simulink model "pmsm_foc_tune_2_2019"  (R2019b)
settings: Solver=VariableStepAuto  StartTime=0.0  StopTime=3  RelTol=1e-3
undefined symbols (not defined in the file): powergui
libraries: simulink x8, eePwmGenerator x6, powerlib x3
settings Model: Creator=ayanc  LastModifiedBy=ayanc

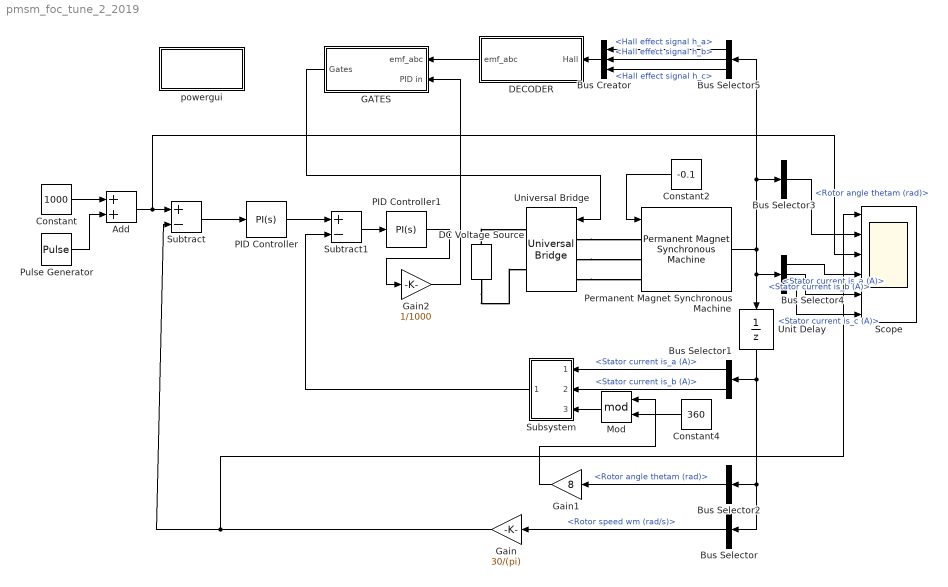
== system pmsm_foc_tune_2_2019 ==
  Add : Sum
  Bus Creator : BusCreator  Inputs=3
  Bus Selector : BusSelector  OutputSignals=Rotor speed wm (rad/s)
  Bus Selector1 : BusSelector  OutputSignals=Stator current is_a (A),Stator current is_b (A)
  Bus Selector2 : BusSelector  OutputSignals=Rotor angle thetam (rad)
  Bus Selector3 : BusSelector  OutputSignals=Rotor angle thetam (rad)
  Bus Selector4 : BusSelector  OutputSignals=Stator current is_a (A),Stator current is_b (A),Stator current is_c (A)
  Bus Selector5 : BusSelector  OutputSignals=Hall effect signal h_a,Hall effect signal h_b,Hall effect signal h_c
  Constant : Constant  Value=1000
  Constant2 : Constant  Value=-0.1
  Constant4 : Constant  Value=360
  DC Voltage Source : powerlib/Electrical Sources/DC Voltage Source  Amplitude=18  Measurements=None
  DECODER : Subsystem
  GATES : Subsystem
  Gain : Gain  Gain=30/(pi)
  Gain1 : Gain  Gain=8
  Gain2 : Gain  Gain=1/1000
  Mod : Math  Operator=mod  SaturateOnIntegerOverflow=on
  PID Controller : simulink/Continuous/PID Controller  Controller=PI  Form=Parallel  TimeDomain=Continuous-time  SampleTime=-1  IntegratorMethod=Forward Euler  FilterMethod=Forward Euler  ControllerParametersSource=internal  P=0.1  I=10  D=0  UseFilter=on  N=100  TunerSelectOption=Transfer Function Based (PID Tuner App)  InitialConditionSource=internal  InitialConditionForIntegrator=0  InitialConditionForFilter=0  DifferentiatorICPrevScaledInput=0  ExternalReset=none  TrackingMode=off  Kt=1  LimitOutput=off  UpperSaturationLimit=18  LowerSaturationLimit=0  LinearizeAsGain=on  AntiWindupMode=none  Kb=1  POutMin=[]  POutMax=[]  IOutMin=[]  IOutMax=[]  DOutMin=[]  DOutMax=[]  NOutMin=[]  NOutMax=[]  SumOutMin=[]  SumOutMax=[]  SaturationOutMin=[]  SaturationOutMax=[]  PParamMin=[]  PParamMax=[]  IParamMin=[]  IParamMax=[]  DParamMin=[]  DParamMax=[]  NParamMin=[]  NParamMax=[]  KbParamMin=[]  KbParamMax=[]  KtParamMin=[]  KtParamMax=[]  KbOutMin=[]  KbOutMax=[]  KtOutMin=[]  KtOutMax=[]  IntegratorOutMin=[]  IntegratorOutMax=[]  FilterOutMin=[]  FilterOutMax=[]  SumI1OutMin=[]  SumI1OutMax=[]  SumI2OutMin=[]  SumI2OutMax=[]  SumI3OutMin=[]  SumI3OutMax=[]  SumI4OutMin=[]  SumI4OutMax=[]  SumDOutMin=[]  SumDOutMax=[]  DifferentiatorOutMin=[]  DifferentiatorOutMax=[]  FilterDiffOutCoefMin=[]  FilterDiffOutCoefMax=[]  ReciprocalOutMin=[]  ReciprocalOutMax=[]  SumDenOutMin=[]  SumDenOutMax=[]  SumNumOutMin=[]  SumNumOutMax=[]  DivideOutMin=[]  DivideOutMax=[]  IntegratorContinuousStateAttributes=''  IntegratorStateMustResolveToSignalObject=off  IntegratorRTWStateStorageClass=Auto  FilterContinuousStateAttributes=''  FilterStateMustResolveToSignalObject=off  FilterRTWStateStorageClass=Auto  ParallelPVariant=InternalParameters  IdealPVariant=Disabled  IVariant=InternalParameters  DVariant=Disabled  IntegratorVariant=Continuous  SatVariant=Disabled  AWVariant=Passthrough  PCopyVariant=Disabled  TRVariant=Disabled  FdbkBlocksVariant=Forward  IdealPFdbkVariant=Disabled  SatFdbkVariant=Disabled  DerivativeFilterVariant=Disabled  NVariant=Disabled  NCopyVariant=Disabled_SignalSpec  FilterICVariant=Disabled  IntegratorICVariant=InternalICs  ExternalResetVariant=Disabled  TRSumVariant=Passthrough  SumFdbkVariant=Disabled  SumVariant=Sum_PI
  PID Controller1 : simulink/Continuous/PID Controller  Controller=PI  Form=Parallel  TimeDomain=Continuous-time  SampleTime=-1  IntegratorMethod=Forward Euler  FilterMethod=Forward Euler  ControllerParametersSource=internal  P=10  I=100  D=0  UseFilter=on  N=100  TunerSelectOption=Transfer Function Based (PID Tuner App)  InitialConditionSource=internal  InitialConditionForIntegrator=0  InitialConditionForFilter=0  DifferentiatorICPrevScaledInput=0  ExternalReset=none  TrackingMode=off  Kt=1  LimitOutput=on  UpperSaturationLimit=1000  LowerSaturationLimit=0  LinearizeAsGain=on  AntiWindupMode=none  Kb=1  POutMin=[]  POutMax=[]  IOutMin=[]  IOutMax=[]  DOutMin=[]  DOutMax=[]  NOutMin=[]  NOutMax=[]  SumOutMin=[]  SumOutMax=[]  SaturationOutMin=[]  SaturationOutMax=[]  PParamMin=[]  PParamMax=[]  IParamMin=[]  IParamMax=[]  DParamMin=[]  DParamMax=[]  NParamMin=[]  NParamMax=[]  KbParamMin=[]  KbParamMax=[]  KtParamMin=[]  KtParamMax=[]  KbOutMin=[]  KbOutMax=[]  KtOutMin=[]  KtOutMax=[]  IntegratorOutMin=[]  IntegratorOutMax=[]  FilterOutMin=[]  FilterOutMax=[]  SumI1OutMin=[]  SumI1OutMax=[]  SumI2OutMin=[]  SumI2OutMax=[]  SumI3OutMin=[]  SumI3OutMax=[]  SumI4OutMin=[]  SumI4OutMax=[]  SumDOutMin=[]  SumDOutMax=[]  DifferentiatorOutMin=[]  DifferentiatorOutMax=[]  FilterDiffOutCoefMin=[]  FilterDiffOutCoefMax=[]  ReciprocalOutMin=[]  ReciprocalOutMax=[]  SumDenOutMin=[]  SumDenOutMax=[]  SumNumOutMin=[]  SumNumOutMax=[]  DivideOutMin=[]  DivideOutMax=[]  IntegratorContinuousStateAttributes=''  IntegratorStateMustResolveToSignalObject=off  IntegratorRTWStateStorageClass=Auto  FilterContinuousStateAttributes=''  FilterStateMustResolveToSignalObject=off  FilterRTWStateStorageClass=Auto  ParallelPVariant=InternalParameters  IdealPVariant=Disabled  IVariant=InternalParameters  DVariant=Disabled  IntegratorVariant=Continuous  SatVariant=Enabled  AWVariant=Passthrough  PCopyVariant=Disabled  TRVariant=Disabled  FdbkBlocksVariant=Forward  IdealPFdbkVariant=Disabled  SatFdbkVariant=Disabled  DerivativeFilterVariant=Disabled  NVariant=Disabled  NCopyVariant=Disabled_SignalSpec  FilterICVariant=Disabled  IntegratorICVariant=InternalICs  ExternalResetVariant=Disabled  TRSumVariant=Passthrough  SumFdbkVariant=Disabled  SumVariant=Sum_PI
  Permanent Magnet Synchronous Machine : powerlib/Machines/Permanent Magnet Synchronous Machine  NbPhases=3  FluxDistribution=Trapezoidal  RotorType=Round  MechanicalLoad=Torque Tm  PresetModel=No  ShowDetailedParameters=on  MeasurementBus=off  Resistance=0.515  Inductance=0.000286  dqInductances=[8.5e-3,8.5e-3]  La=0.000286  MachineConstant=Flux linkage established by magnets (V.s)  Flux=0.00341897  VoltageCst=5.7285  TorqueCst=0.054704  Flat=120  Mechanical=[1.35e-05 0.00108862 8]  PolePairs=4  InitialConditions=[0,0, 0,0]  InitialConditions5ph=[0 0 0 0 0 0]  RefAngle=90 degrees behind phase A axis (modified Park)  IterativeDiscreteModel=Trapezoidal non iterative  TsBlock=-1  TsPowergui=0
  Pulse Generator : DiscretePulseGenerator  PulseType=Time based  Amplitude=500  Period=1.5  PulseWidth=50
  Scope : Scope  NumInputPorts=6
  Subsystem : Subsystem
  Subtract : Sum  Inputs=+-
  Subtract1 : Sum  Inputs=+-
  Unit Delay : UnitDelay  SampleTime=10e-6  HasFrameUpgradeWarning=on
  Universal Bridge : powerlib/Power Electronics/Universal Bridge  Arms=3  SnubberResistance=1e5  SnubberCapacitance=inf  Device=MOSFET / Diodes  Ron=1e-3  Lon=0  ForwardVoltages="[  0  0  ]"  ForwardVoltage=0  GTOparameters=[ 10e-6 , 20e-6 ]  IGBTparameters=[ 1e-6 , 2e-6 ]  Measurements=None  Measurements_2=None  converterType=Rectifier
  powergui : Subsystem  Priority=1  AncestorBlock=powerlib/powergui  DialogController=POWERSYS.PowerSysDialog  InitFcn=powergui( 'InitFcn_Callback' , gcb , 0 , [ ] );  mask(PSB option menu block){SimulationMode=Continuous, SampleTime=50e-6, frequency=60, Iterations=50, frequencyindice=0, Pbase=100e6, ErrMax=1e-4, UnitsV=kV, UnitsW=MW, buscounter=0, FunctionMessages=off, echomessages=off, EnableUseOfTLC=off, CurrentSourceSwitches=off, DisableSnubberDevices=off, DisableRonSwitches=off, DisableVfSwitches=off, DisplayEquations=off, AutomaticDiscreteSolvers=off, SolverType=Tustin/Backward Euler (TBE), Interpol=off, ExternalGateDelay=off, methode=off, Ts=100, x0status=blocks, SPID=on, SwTol=0, HookPort=off, NonlinearTolerance=1e-4, nMaxIteration=100, ContinueOnMaxIteration=off, RestoreLinks=warning, ResistiveCurrentMeasurement=off, Frange=[0:2:500], Ylog=off, Xlog=on, ShowGrid=off, save=off, variable=ZData, structure=0, ZoomFFT=off, StartTime=0.0, cycles=1, DisplayStyle=1, fundamental=60, FreqAxis=off, MaxFrequency=1000, frequencyindicesteady=1, RmsSteady=1, display=off}
      mask prompts: SimulationMode "Simulation type:"; SampleTime "Sample time (s):"; frequency "Frequency (Hz):"; Iterations "Max iterations"; frequencyindice "Frequency (Hz)"; Pbase "Base power (VA)"; ErrMax "PQ tolerance (pu)"; UnitsV "Voltage units"; UnitsW "Power units"; buscounter "Load flow bus counter"; FunctionMessages "Disable Specialized Power Systems warnings"; echomessages "Display Specialized Power Systems compilation messages"; EnableUseOfTLC "Use TLC file when in Accelerator Simulation Mode and for code generation"; CurrentSourceSwitches "Disable ideal switching"; DisableSnubberDevices "Disable snubbers in switching devices"; DisableRonSwitches "Disable Ron resistances in switching devices"; DisableVfSwitches "Disable forward voltages in switching devices"; DisplayEquations "Display circuit differential equations"; AutomaticDiscreteSolvers "Automatically handle Discrete solver and Advanced tab solver settings of blocks"; SolverType "Discrete solver"; Interpol "Interpolate switching events"; ExternalGateDelay "Use time-stamped gate signals"; methode "Store switching topologies"; Ts "Buffer size (MBytes):"; x0status "Start simulation with initial electrical states from:"; SPID "Use ideal switching devices"; SwTol "Switch tolerance"; HookPort "Allow multiple powergui blocks"; NonlinearTolerance "Solver tolerance"; nMaxIteration "Maximum number of iterations"; ContinueOnMaxIteration "Continue Simulation if maximum number of iterations is reached"; RestoreLinks "Restore disabled links of Simscape Power Systems ST blocks:"; ResistiveCurrentMeasurement "Use non ideal current measurement blocks (1e-4Ohm internal resistance)"; Frange "Frequency Range"; Ylog "Log impedance"; Xlog "log Frequency"; ShowGrid "grid"; save "Save Data To Workspace"; variable "Variable Name"; structure "Structure Name (PSBFFTSCOPE)"; ZoomFFT "ZoomFFT (PSBFFTSCOPE)"; StartTime "Start Time (PSBFFTSCOPE)"; cycles "Cycles (PSBFFTSCOPE)"; DisplayStyle "Display style (PSBFFTSCOPE)"; fundamental "Fundamental (PSBFFTSCOPE)"; FreqAxis "Frequency Axis (PSBFFTSCOPE)"; MaxFrequency "Max Frequency (PSBFFTSCOPE)"; frequencyindicesteady "Frequency indice (STEADYSTATE)"; RmsSteady "RMS display (STEADYSTATE)"; display "Display Results"
      mask help: Set simulation type, simulation parameters, and preferences.
      mask init:
      | dispMessage = powergui('MaskInitialization',gcb,SimulationMode,SampleTime);
      settings: PreSaveFcn=powergui( 'PreSaveFcn_Callback' , gcb , [ ] , [ ] );  OpenFcn=sps_rtmsupport('OpenFcn',gcbh)
      mask Help: helpview(psbhelp)
      mask TypeOptions SimulationMode: Continuous | Discrete | Phasor | Discrete phasor
      mask Callback SimulationMode: powergui('SimulationType',[],[],gcb);
      mask TypeOptions UnitsV: V | kV
      mask TypeOptions UnitsW: W | kW | MW
      mask Callback CurrentSourceSwitches: powergui('SimulationType',[],[],gcb);
      mask Callback AutomaticDiscreteSolvers: powergui('SimulationType',[],[],gcb);
      mask TypeOptions SolverType: Tustin/Backward Euler (TBE) | Tustin | Backward Euler
      mask Callback SolverType: powergui('SimulationType',[],[],gcb);
      mask Callback Interpol: powergui('SimulationType',[],[],gcb);
      mask Callback ExternalGateDelay: powergui('SimulationType',[],[],gcb);
      mask Callback methode: powergui('SimulationType',[],[],gcb);
      mask TypeOptions x0status: blocks | steady | zero
      mask TypeOptions RestoreLinks: yes | warning | no
      mask Callback display: sps_rtmsupport('parametereditingmodes',gcbh) % Will be executed last in parameter callbacks to ensure mask enable consistency
      mask DialogControl SolverTab Prompt: Solver
      mask DialogControl AutoSolverNote Prompt: The Simulation type parameter is governed by Simulink. To access the Powergui solver settings, unselect auto (Automatic solver selection) solver in the Simulink solver options.
      mask DialogControl AnalysisTools Prompt: Tools
      mask DialogControl SteadyState Prompt: Steady-State
      mask DialogControl SteadyState Callback:
      | close_system(gcb)
      | power_steadystate(bdroot(gcb),gcb);
      mask DialogControl InitialState Prompt: Initial State
      mask DialogControl InitialState Callback:
      | close_system(gcb)
      | power_initstates(bdroot(gcb),gcb)
      mask DialogControl MachineInitialization Prompt: Machine Initialization
      mask DialogControl MachineInitialization Callback:
      | close_system(gcb)
      | power_loadflow(bdroot(gcb),gcb)
      mask DialogControl ImpedanceMeasurement Prompt: Impedance Measurement
      mask DialogControl ImpedanceMeasurement Callback:
      | close_system(gcb)
      | power_zmeter(bdroot(gcb),gcb)
      mask DialogControl FFTAnalysis Prompt: FFT Analysis
      mask DialogControl FFTAnalysis Callback:
      | close_system(gcb)
      | power_fftscope(bdroot(gcb),gcb)
      mask DialogControl LinearSystemAnalyzer Prompt: Use Linear System Analyzer
      mask DialogControl LinearSystemAnalyzer Callback:
      | close_system(gcb)
      | power_ltiview(bdroot(gcb),gcb)
      mask DialogControl HysteresisDesign Prompt: Hysteresis Design
      mask DialogControl HysteresisDesign Callback:
      | close_system(gcb)
      | power_hysteresis(bdroot(gcb),gcb)
      mask DialogControl RLCLineParameters Prompt: RLC Line Parameters
      mask DialogControl RLCLineParameters Callback:
      | close_system(gcb)
      | power_lineparam(bdroot(gcb),gcb)
      mask DialogControl GenerateReprot Prompt: Generate Report
      mask DialogControl GenerateReprot Callback:
      | close_system(gcb)
      | power_report(bdroot(gcb),gcb)
      mask DialogControl Control14 Prompt: Customize SPS blocks
      mask DialogControl Control14 Callback:
      | close_system(gcb);
      | power_customize;
      mask DialogControl LoadFlow Prompt: Load Flow
      mask DialogControl LoadFlow Callback:
      | close_system(gcb)
      | power_loadflow('-v2',bdroot(gcb))
      mask DialogControl Container14 Prompt: Load flow settings
      mask DialogControl ParameterTabVar012 Prompt: Preferences
      mask DialogControl Solver Prompt: Solver
      mask DialogControl SolverDetails Prompt: Solver details for nonlinear elements
      mask Display: color('blue'),disp(dispMessage)
  wires:
  Gain/1 -> Scope/1, Subtract/2
  Subtract/1 -> PID Controller/1
  PID Controller/1 -> Subtract1/1
  Bus Selector2/1 -> Gain1/1  "<Rotor angle thetam (rad)>"
  Gain1/1 -> Mod/1
  Subtract1/1 -> PID Controller1/1
  Bus Selector3/1 -> Scope/2  "<Rotor angle thetam (rad)>"
  Bus Selector/1 -> Gain/1  "<Rotor speed wm (rad/s)>"
  Unit Delay/1 -> Bus Selector2/1, Bus Selector/1, Bus Selector1/1
  Bus Selector4/1 -> Scope/4  "<Stator current is_a (A)>"
  Bus Selector4/2 -> Scope/5  "<Stator current is_b (A)>"
  Bus Selector4/3 -> Scope/6  "<Stator current is_c (A)>"
  Constant2/1 -> Permanent Magnet Synchronous Machine/1
  Bus Selector1/2 -> Subsystem/2(In1)  "<Stator current is_b (A)>"
  Bus Selector1/1 -> Subsystem/1(In2)  "<Stator current is_a (A)>"
  Mod/1 -> Subsystem/3(In3)
  Constant4/1 -> Mod/2
  Bus Selector5/3 -> Bus Creator/3  "<Hall effect signal h_c>"
  Permanent Magnet Synchronous Machine/1 -> Bus Selector4/1, Unit Delay/1, Bus Selector5/1, Bus Selector3/1
  Bus Creator/1 -> DECODER/1("Hall ")
  Bus Selector5/2 -> Bus Creator/2  "<Hall effect signal h_b>"
  Bus Selector5/1 -> Bus Creator/1  "<Hall effect signal h_a>"
  DECODER/1(emf_abc) -> GATES/1("emf_abc ")
  GATES/1(Gates) -> Universal Bridge/1
  Subsystem/1(Out1) -> Subtract1/2
  Constant/1 -> Add/1
  Pulse Generator/1 -> Add/2
  Add/1 -> Scope/3, Subtract/1
  Gain2/1 -> GATES/2("PID in ")
  PID Controller1/1 -> Gain2/1
  connections:
  DC Voltage Source/LConn1 -- Universal Bridge/RConn2
  DC Voltage Source/RConn1 -- Universal Bridge/RConn1
  Universal Bridge/LConn1 -- Permanent Magnet Synchronous Machine/LConn1
  Universal Bridge/LConn2 -- Permanent Magnet Synchronous Machine/LConn2
  Universal Bridge/LConn3 -- Permanent Magnet Synchronous Machine/LConn3

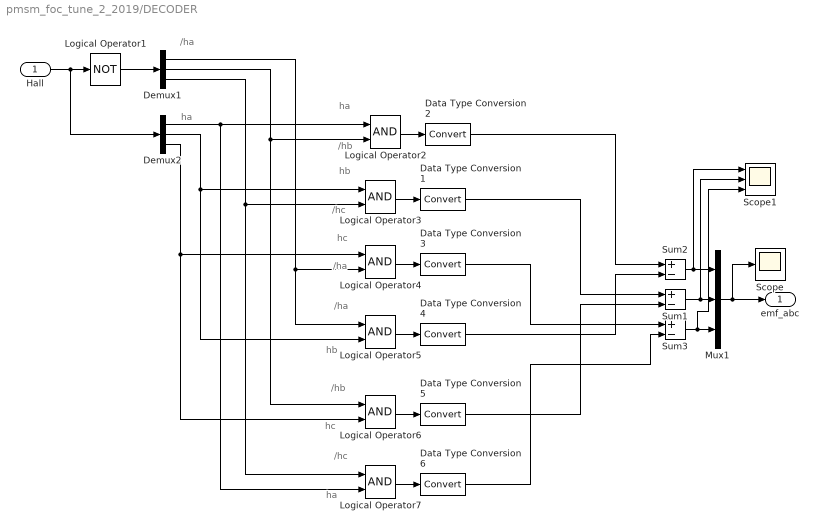
== system pmsm_foc_tune_2_2019/DECODER ==
  note: hc
  note: ha
  note: /ha
  note: hb
  note: hb
  note: /hb
  note: /hb
  note: /ha
  note: /hc
  note: ha
  note: /ha
  note: /hc
  note: hc
  note: ha
  "Hall " : Inport
  Data Type Conversion{1..6} (6 alike) : DataTypeConversion
  Demux1 : Demux  Outputs=3
  Demux2 : Demux  Outputs=3
  Logical Operator1 : Logic  Operator=NOT  AllPortsSameDT=off  OutDataTypeStr=boolean
  Logical Operator{2..7} (6 alike) : Logic  AllPortsSameDT=off  OutDataTypeStr=boolean
  Mux1 : Mux  Inputs=3
  Scope : Scope
  Scope1 : Scope  NumInputPorts=3
  Sum1 : Sum  Inputs=+-  OutDataTypeStr=double
  Sum2 : Sum  Inputs=+-  OutDataTypeStr=double
  Sum3 : Sum  Inputs=+-  OutDataTypeStr=double
  emf_abc : Outport  VectorParamsAs1DForOutWhenUnconnected=off
  wires:
  Data Type Conversion2/1 -> Sum2/1
  Data Type Conversion3/1 -> Sum3/1
  Logical Operator5/1 -> Data Type Conversion4/1
  Mux1/1 -> Scope/1, emf_abc/1
  Logical Operator2/1 -> Data Type Conversion2/1
  Data Type Conversion1/1 -> Sum1/1
  Data Type Conversion4/1 -> Sum2/2
  Demux1/1 -> Logical Operator4/2, Logical Operator5/1
  Data Type Conversion6/1 -> Sum3/2
  Demux2/2 -> Logical Operator3/1, Logical Operator5/2
  Data Type Conversion5/1 -> Sum1/2
  Logical Operator1/1 -> Demux1/1
  "Hall "/1 -> Logical Operator1/1, Demux2/1
  Logical Operator4/1 -> Data Type Conversion3/1
  Logical Operator6/1 -> Data Type Conversion5/1
  Demux2/1 -> Logical Operator2/1, Logical Operator7/2
  Logical Operator3/1 -> Data Type Conversion1/1
  Demux2/3 -> Logical Operator4/1, Logical Operator6/2
  Logical Operator7/1 -> Data Type Conversion6/1
  Demux1/2 -> Logical Operator2/2, Logical Operator6/1
  Sum1/1 -> Scope1/2, Mux1/2
  Demux1/3 -> Logical Operator3/2, Logical Operator7/1
  Sum2/1 -> Scope1/1, Mux1/1
  Sum3/1 -> Scope1/3, Mux1/3

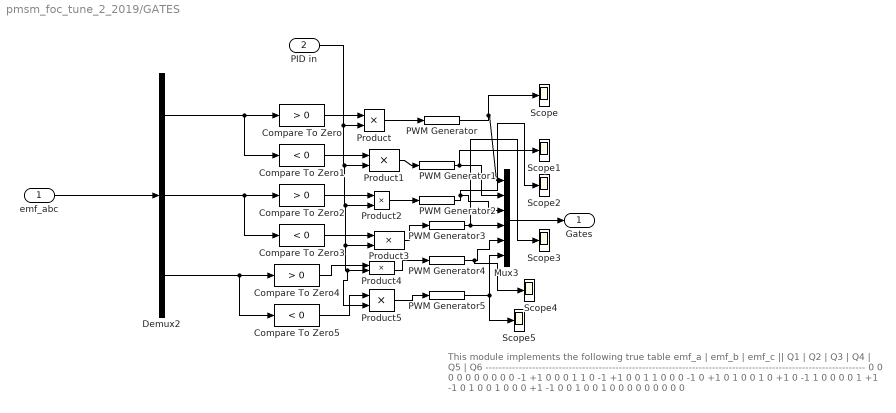
== system pmsm_foc_tune_2_2019/GATES ==
  note: This module implements the following true table
      |
      |    emf_a   |   emf_b   |   emf_c   ||   Q1   |   Q2   |   Q3   |   Q4   |   Q5   |   Q6
      |     ------------------------------------------------------------------------------------------------------------------
      |       0              0                0            0          0          0           0        0        0
      |       0               -1              +1          0          0          0           1        1        0
      |     -1              +1                0          0          1          1           0        0        0
      |     -1               0               +1          0          1         0           0        1        0
      |    +1               0                -1          1          0          0           0        0        1
      |    +1              -1                0           1          0          0           1        0        0
      |      0              +1               -1           0          0          1           0        0        1
      |     0              0                0             0          0          0           0        0        0
  "emf_abc " : Inport
  "PID in " : Inport  Port=2
  Compare To Zero : simulink/Logic and Bit Operations/Compare To Zero  relop=>  OutDataTypeStr=boolean  ZeroCross=off
  Compare To Zero1 : simulink/Logic and Bit Operations/Compare To Zero  relop=<  OutDataTypeStr=boolean  ZeroCross=off
  Compare To Zero2 : simulink/Logic and Bit Operations/Compare To Zero  relop=>  OutDataTypeStr=boolean  ZeroCross=off
  Compare To Zero3 : simulink/Logic and Bit Operations/Compare To Zero  relop=<  OutDataTypeStr=boolean  ZeroCross=off
  Compare To Zero4 : simulink/Logic and Bit Operations/Compare To Zero  relop=>  OutDataTypeStr=boolean  ZeroCross=off
  Compare To Zero5 : simulink/Logic and Bit Operations/Compare To Zero  relop=<  OutDataTypeStr=boolean  ZeroCross=off
  Demux2 : Demux  Outputs=3
  Mux3 : Mux  Inputs=6
  PWM Generator{,1..5} (6 alike) : eePwmGenerator/PWM Generator  CarrCount=Up  Tper=1e-04  Ts=0
  Product{,1..5} (6 alike) : Product
  Scope{,1..5} (6 alike) : Scope
  Gates : Outport  VectorParamsAs1DForOutWhenUnconnected=off
  wires:
  Compare To Zero4/1 -> Product4/1
  Product1/1 -> PWM Generator1/1
  "PID in "/1 -> Product5/2, Product4/2, Product3/2, Product2/2, Product1/2, Product/2
  Demux2/2 -> Compare To Zero2/1, Compare To Zero3/1
  PWM Generator5/1 -> Scope5/1, Mux3/6
  PWM Generator3/1 -> Mux3/4, Scope3/1
  Product5/1 -> PWM Generator5/1
  Compare To Zero3/1 -> Product3/1
  PWM Generator2/1 -> Scope2/1, Mux3/3
  Product3/1 -> PWM Generator3/1
  "emf_abc "/1 -> Demux2/1
  Mux3/1 -> Gates/1
  Product4/1 -> PWM Generator4/1
  Compare To Zero1/1 -> Product1/1
  PWM Generator4/1 -> Scope4/1, Mux3/5
  Demux2/3 -> Compare To Zero4/1, Compare To Zero5/1
  Compare To Zero/1 -> Product/1
  Product2/1 -> PWM Generator2/1
  Product/1 -> PWM Generator/1
  Compare To Zero5/1 -> Product5/1
  Demux2/1 -> Compare To Zero/1, Compare To Zero1/1
  PWM Generator/1 -> Scope/1, Mux3/1
  PWM Generator1/1 -> Scope1/1, Mux3/2
  Compare To Zero2/1 -> Product2/1

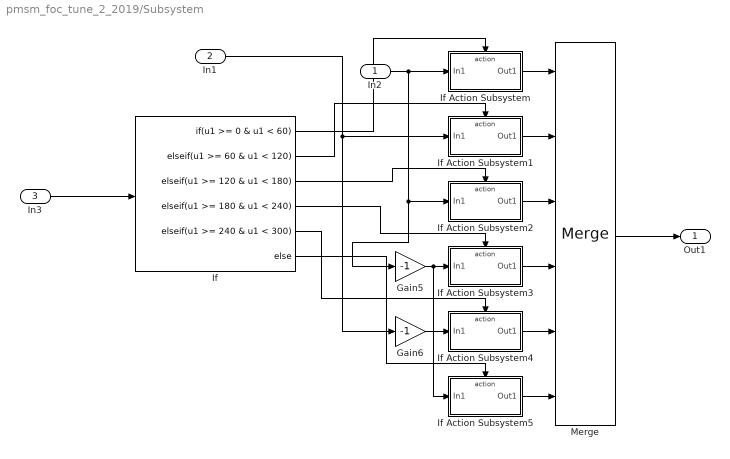
== system pmsm_foc_tune_2_2019/Subsystem ==
  In2 : Inport
  In1 : Inport  Port=2
  In3 : Inport  Port=3
  Gain5 : Gain  Gain=-1
  Gain6 : Gain  Gain=-1
  If : If  IfExpression=u1 >= 0 & u1 < 60  ElseIfExpressions=u1 >= 60 & u1 < 120, u1 >= 120 & u1 < 180, u1 >= 180 & u1 < 240, u1 >= 240 & u1 < 300
  If Action Subsystem : Subsystem  TreatAsAtomicUnit=on
  If Action Subsystem1 : Subsystem  TreatAsAtomicUnit=on
  If Action Subsystem2 : Subsystem  TreatAsAtomicUnit=on
  If Action Subsystem3 : Subsystem  TreatAsAtomicUnit=on
  If Action Subsystem4 : Subsystem  TreatAsAtomicUnit=on
  If Action Subsystem5 : Subsystem  TreatAsAtomicUnit=on
  Merge : Merge  Inputs=6
  Out1 : Outport
  wires:
  If Action Subsystem/1(Out1) -> Merge/1
  Gain5/1 -> If Action Subsystem5/1(In1), If Action Subsystem3/1(In1)
  If Action Subsystem3/1(Out1) -> Merge/4
  If Action Subsystem5/1(Out1) -> Merge/6
  In2/1 -> Gain5/1, If Action Subsystem2/1(In1), If Action Subsystem/1(In1)
  In1/1 -> Gain6/1, If Action Subsystem1/1(In1)
  If/6 -> If Action Subsystem5/Action
  If Action Subsystem4/1(Out1) -> Merge/5
  If Action Subsystem1/1(Out1) -> Merge/2
  If/3 -> If Action Subsystem2/Action
  If/2 -> If Action Subsystem1/Action
  If/4 -> If Action Subsystem3/Action
  If/1 -> If Action Subsystem/Action
  If Action Subsystem2/1(Out1) -> Merge/3
  Gain6/1 -> If Action Subsystem4/1(In1)
  If/5 -> If Action Subsystem4/Action
  In3/1 -> If/1
  Merge/1 -> Out1/1

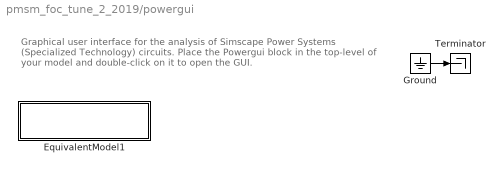
== system pmsm_foc_tune_2_2019/powergui ==
  note: Graphical user interface for the analysis of
      | Simscape Power Systems (Specialized Technology) circuits.
      | Place the Powergui block in the top-level of your model and double-click
      | on it to open the GUI.
  EquivalentModel1 : Subsystem  mask{SwTol=0}
      mask prompts: SwTol "SwitchTolerance"
      mask init:
      | S  = GetDataForEquivalentModel('SPID',gcbh,SwTol);
      mask Display:
      | color('blue')
      | disp('EQUIVALENT CIRCUIT\nSPID')
  Ground : Ground
  Terminator : Terminator
  wires:
  Ground/1 -> Terminator/1

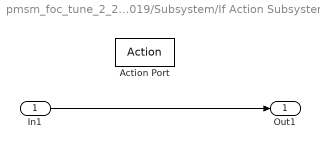
== system pmsm_foc_tune_2_2019/Subsystem/If Action Subsystem ==
  In1 : Inport
  Action Port : ActionPort  ActionPortLabel=if(u1 >= 0 & u1 < 60)
  Out1 : Outport
  wires:
  In1/1 -> Out1/1

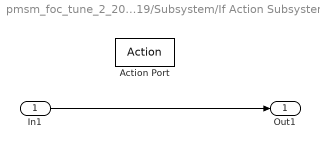
== system pmsm_foc_tune_2_2019/Subsystem/If Action Subsystem1 ==
  In1 : Inport
  Action Port : ActionPort  ActionPortLabel=elseif(u1 >= 60 & u1 < 120)
  Out1 : Outport
  wires:
  In1/1 -> Out1/1

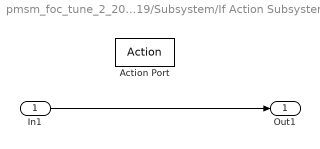
== system pmsm_foc_tune_2_2019/Subsystem/If Action Subsystem2 ==
  In1 : Inport
  Action Port : ActionPort  ActionPortLabel=elseif( u1 >= 120 & u1 < 180)
  Out1 : Outport
  wires:
  In1/1 -> Out1/1

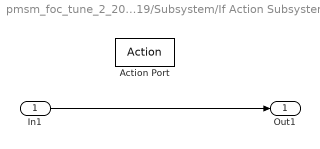
== system pmsm_foc_tune_2_2019/Subsystem/If Action Subsystem3 ==
  In1 : Inport
  Action Port : ActionPort  ActionPortLabel=elseif( u1 >= 180 & u1 < 240)
  Out1 : Outport
  wires:
  In1/1 -> Out1/1

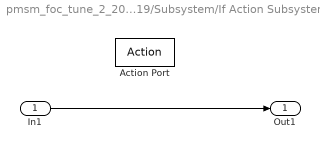
== system pmsm_foc_tune_2_2019/Subsystem/If Action Subsystem4 ==
  In1 : Inport
  Action Port : ActionPort  ActionPortLabel=elseif( u1 >= 240 & u1 < 300)
  Out1 : Outport
  wires:
  In1/1 -> Out1/1

== system pmsm_foc_tune_2_2019/Subsystem/If Action Subsystem5 ==
  In1 : Inport
  Action Port : ActionPort  ActionPortLabel=else
  Out1 : Outport
  wires:
  In1/1 -> Out1/1

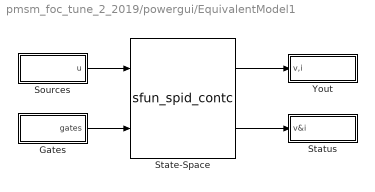
== system pmsm_foc_tune_2_2019/powergui/EquivalentModel1 ==
  Gates : Subsystem
  Sources : Subsystem
  State-Space : S-Function  FunctionName=sfun_spid_contc  Parameters=S.Mg, [S.nb.x S.nb.u S.nb.y S.nb.s], S.x0, S.MgColNames, S.SwitchVf, S.SwitchType, S.SwitchGateInitialValue, S.SwitchTolerance,S.SaveMatrices,S.BufferSize  SFunctionDeploymentMode=off  EnableBusSupport=off
  Status : Subsystem
  Yout : Subsystem
  wires:
  State-Space/1 -> Yout/1(v,i)
  State-Space/2 -> Status/1(v&i)
  Sources/1(u) -> State-Space/1
  Gates/1(gates) -> State-Space/2

== system pmsm_foc_tune_2_2019/powergui/EquivalentModel1/Gates ==
  Mux : Mux  Inputs=1
  gates : Outport  VectorParamsAs1DForOutWhenUnconnected=off
  wires:
  Mux/1 -> gates/1
  [T37_3613_2226342085195] -> Mux/1

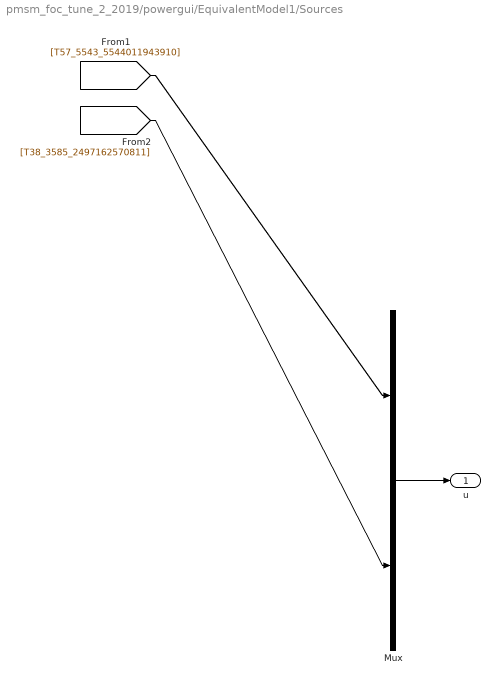
== system pmsm_foc_tune_2_2019/powergui/EquivalentModel1/Sources ==
  Mux : Mux  Inputs=[2 1]
  u : Outport  VectorParamsAs1DForOutWhenUnconnected=off
  wires:
  Mux/1 -> u/1
  [T57_5543_5544011943910] -> Mux/1
  [T38_3585_2497162570811] -> Mux/2

== system pmsm_foc_tune_2_2019/powergui/EquivalentModel1/Status ==
  v&i : Inport
  Demux : Demux  Outputs=1
  tag scope: T39_3848_2680141846491=global
  wires:
  v&i/1 -> Demux/1
  Demux/1 -> [T39_3848_2680141846491]

== system pmsm_foc_tune_2_2019/powergui/EquivalentModel1/Yout ==
  v,i : Inport
  Demux : Demux  Outputs=1
  tag scope: T57_5538_5490517260514=global
  wires:
  v,i/1 -> Demux/1
  Demux/1 -> [T57_5538_5490517260514]
